simulink library "alfa_ceiling"  (R2018b)
settings: Solver=ode45  StartTime=0.0  StopTime=10.0  RelTol=1e-3  EnableMultiTasking=on
settings Model: Creator=lena.frank  LastModifiedBy=drhf
settings DataIOCC: LimitDataPoints=on  SaveFormat=Array  SignalLoggingSaveFormat=ModelDataLogs
settings OptimizationCC: ExpressionDepthLimit=2147483647  LifeSpan=inf
settings DebuggingCC: UnderspecifiedInitializationDetection=Classic  MergeDetectMultiDrivingBlocksExec=none  SolverPrmCheckMsg=warning  FcnCallInpInsideContextMsg=warning  StateNameClashWarn=warning  SFUnexpectedBacktrackingDiag=warning  SFNoUnconditionalDefaultTransitionDiag=warning  SFExecutionAtInitializationDiag=none
settings HardwareCC: ProdBitPerPointer=32  ProdBitPerSizeT=32  ProdBitPerPtrDiffT=32  ProdLargestAtomicFloat=None  ProdIntDivRoundTo=Undefined  ProdEndianess=Unspecified  ProdWordSize=32  ProdHWDeviceType=32-bit Generic
settings ModelReferenceCC: PropagateSignalLabelsOutOfModel=off
settings SFSimCC: SimUseLocalCustomCode=off
settings RTWCC: RTWUseLocalCustomCode=off
settings CodeAppCC: StateflowObjectComments=on
settings GRTTargetCC: TargetLangStandard=C89/C90 (ANSI)  GeneratePreprocessorConditionals=Disable all  CombineOutputUpdateFcns=off  GRTInterface=on
settings ConfigComp: CovMetricSettings=dw  CovHtmlReporting=on  CovSaveCumulativeToWorkspaceVar=on  CovSaveSingleToWorkspaceVar=on  CovExternalEMLEnable=off

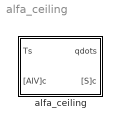
== system alfa_ceiling ==
  alfa_ceiling : Subsystem  mask(ALFA){active=0, emission_c=0.65, wallsurface=1}
      mask prompts: active "active layer (0 / 1)"; emission_c "Longwave emissivity of surface (0..1)"; wallsurface "Ceiling surface in m²"
      mask help:
      | Convective and radiative heat transfer at the SURFACE OF A HORIZONTAL CEELING.
      | [AIV] : conditions of zone node,
      | Ts : temperature of outdoor wall surface, °C,
      | qdots : specific heat flow into wall construction, W/m^2,
      | [S] : heat and air flow to zone node.
      mask Help: web(fullfile(path_carnot('help'),'alfa_ceiling.html'),'-helpbrowser')

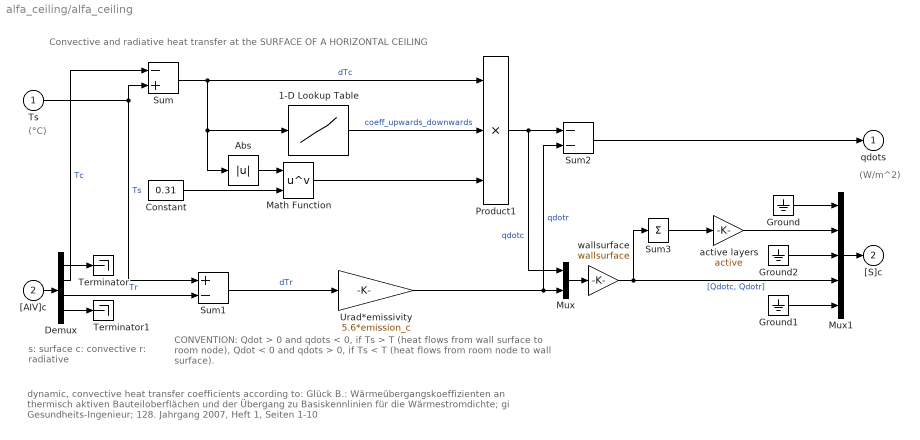
== system alfa_ceiling/alfa_ceiling ==
  note: dynamic, convective heat transfer coefficients according to: Glück B.: Wärmeübergangskoeffizienten an thermisch aktiven Bauteiloberflächen
      | und der Übergang zu Basiskennlinien für die Wärmestromdichte; gi Gesundheits-Ingenieur; 128. Jahrgang 2007, Heft 1, Seiten 1-10
  note: CONVENTION:
      | Qdot > 0 and qdots < 0, if Ts > T (heat flows from wall surface to room node),
      | Qdot < 0 and qdots > 0, if Ts < T (heat flows from room node to wall surface).
  note: s: surface
      | c: convective
      | r: radiative
  note: Convective and radiative heat transfer at the SURFACE OF A HORIZONTAL CEILING
  note: (W/m^2)
  note: (°C)
  Ts : Inport
  "[AIV]c" : Inport  Port=2
  1-D Lookup Table : Lookup_n-D  NumberOfTableDimensions=1  BreakpointsForDimension1=[-10 -0.01 0.01 10]  BeginIndexSearchUsingPreviousIndexResult=on  Table=[2 2 0.54 0.54]  InternalRulePriority=Speed  RndMeth=Simplest  InputSameDT=on
  Abs : Abs
  Constant : Constant  Value=0.31
  Demux : Demux  Outputs=[1 1 1 6]
  Ground : Ground
  Ground1 : Ground
  Ground2 : Ground
  Math Function : Math  Operator=pow  SaturateOnIntegerOverflow=on
  Mux : Mux  Inputs=[1 1]
  Mux1 : Mux  Inputs=[4 1 1 2 5]
  Product1 : Product  Inputs=3  SaturateOnIntegerOverflow=on  RndMeth=Zero  InputSameDT=on  OutDataTypeStr=Inherit: Same as first input
  Sum : Sum  Inputs=-+  SaturateOnIntegerOverflow=on  InputSameDT=on  OutDataTypeStr=Inherit: Same as first input
  Sum1 : Sum  Inputs=+-  SaturateOnIntegerOverflow=on  InputSameDT=on  OutDataTypeStr=Inherit: Same as first input
  Sum2 : Sum  Inputs=--  SaturateOnIntegerOverflow=on  InputSameDT=on  OutDataTypeStr=Inherit: Same as first input
  Sum3 : Sum  Inputs=1  SaturateOnIntegerOverflow=on  InputSameDT=on  OutDataTypeStr=Inherit: Same as first input
  Terminator : Terminator
  Terminator1 : Terminator
  Urad*emissivity : Gain  Gain=5.6*emission_c  SaturateOnIntegerOverflow=on  OutDataTypeStr=Inherit: Same as input  ParamDataTypeStr=Inherit: Same as input
  active layers : Gain  Gain=active  SaturateOnIntegerOverflow=on  OutDataTypeStr=Inherit: Same as input  ParamDataTypeStr=Inherit: Same as input
  wallsurface : Gain  Gain=wallsurface  SaturateOnIntegerOverflow=on  OutDataTypeStr=Inherit: Same as input  ParamDataTypeStr=Inherit: Same as input
  qdots : Outport
  "[S]c" : Outport  Port=2
  wires:
  Demux/3 -> Sum1/2  "Tr"
  Sum/1 -> 1-D Lookup Table/1, Abs/1, Product1/1  "dTc"
  Product1/1 -> Mux/1, Sum2/1  "qdotc"
  Sum2/1 -> qdots/1
  Demux/4 -> Terminator1/1
  "[AIV]c"/1 -> Demux/1
  Demux/1 -> Terminator/1
  Sum1/1 -> Urad*emissivity/1  "dTr"
  Urad*emissivity/1 -> Sum2/2, Mux/2  "qdotr"
  Mux/1 -> wallsurface/1
  Demux/2 -> Sum/1  "Tc"
  Ts/1 -> Sum1/1, Sum/2  "Ts"
  wallsurface/1 -> Mux1/4, Sum3/1  "[Qdotc, Qdotr]"
  Sum3/1 -> active layers/1
  Ground/1 -> Mux1/1
  Ground1/1 -> Mux1/5
  Mux1/1 -> "[S]c"/1
  Ground2/1 -> Mux1/3
  active layers/1 -> Mux1/2
  Constant/1 -> Math Function/2
  Abs/1 -> Math Function/1
  1-D Lookup Table/1 -> Product1/2  "coeff_upwards_downwards"
  Math Function/1 -> Product1/3
